simulink model "fen_ut"  (Simulink 8.1)
settings: Solver=FixedStepDiscrete  StartTime=0.0  StopTime=Inf  FixedStep=0.005  RelTol=1e-3
libraries: fen x1
settings Model: Creator=xsellart  LastModifiedBy=AT015555
settings DataIOCC: SignalLoggingSaveFormat=Dataset
settings OptimizationCC: ExpressionDepthLimit=128
settings DebuggingCC: FcnCallInpInsideContextMsg=EnableAllAsError
settings GRTTargetCC: CombineOutputUpdateFcns=on  GRTInterface=off

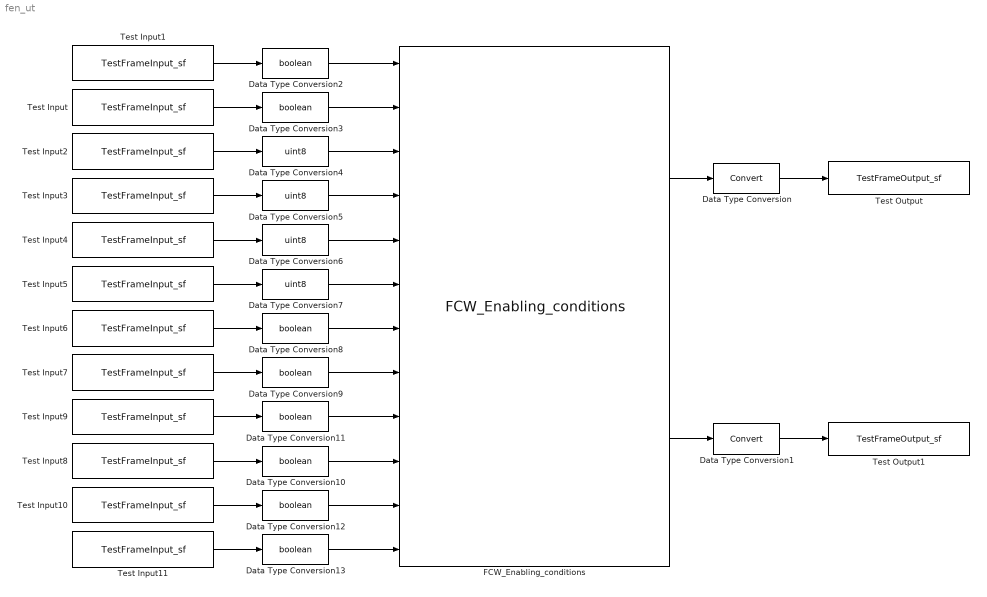
== system fen_ut ==
  Data Type Conversion : DataTypeConversion
  Data Type Conversion1 : DataTypeConversion
  Data Type Conversion{2..3,8..13} (8 alike) : DataTypeConversion  OutDataTypeStr=boolean
  Data Type Conversion{4..7} (4 alike) : DataTypeConversion  OutDataTypeStr=uint8
  FCW_Enabling_conditions : fen/FCW_Enabling_conditions
  Test Input : S-Function  FunctionName=TestFrameInput_sf  Parameters=varname,sampletime  EnableBusSupport=off  mask(Test Input){varname=VDINR_FCWEnableO_flg, sampletime=0.005}
      mask prompts: varname "Name:"; sampletime "Sample Time:"
      mask help: Outputs the value of a Test Input variable from an Excel spreadsheet when used with the runsiltest script. Otherwise outputs 0.
      mask Display: fprintf('Test Input:\n%s',varname);
  Test Input1 : S-Function  FunctionName=TestFrameInput_sf  Parameters=varname,sampletime  EnableBusSupport=off  mask(Test Input){varname=VDINR_FCWEnableH_flg, sampletime=0.005}
      mask prompts: varname "Name:"; sampletime "Sample Time:"
      mask help: Outputs the value of a Test Input variable from an Excel spreadsheet when used with the runsiltest script. Otherwise outputs 0.
      mask Display: fprintf('Test Input:\n%s',varname);
  Test Input10 : S-Function  FunctionName=TestFrameInput_sf  Parameters=varname,sampletime  EnableBusSupport=off  mask(Test Input){varname=VDHP_DisableADASFun_flg, sampletime=0.005}
      mask prompts: varname "Name:"; sampletime "Sample Time:"
      mask help: Outputs the value of a Test Input variable from an Excel spreadsheet when used with the runsiltest script. Otherwise outputs 0.
      mask Display: fprintf('Test Input:\n%s',varname);
  Test Input11 : S-Function  FunctionName=TestFrameInput_sf  Parameters=varname,sampletime  EnableBusSupport=off  mask(Test Input){varname=VDHP_DisableFCW_flg, sampletime=0.005}
      mask prompts: varname "Name:"; sampletime "Sample Time:"
      mask help: Outputs the value of a Test Input variable from an Excel spreadsheet when used with the runsiltest script. Otherwise outputs 0.
      mask Display: fprintf('Test Input:\n%s',varname);
  Test Input2 : S-Function  FunctionName=TestFrameInput_sf  Parameters=varname,sampletime  EnableBusSupport=off  mask(Test Input){varname=VDINR_KeySwitchStatus_enum, sampletime=0.005}
      mask prompts: varname "Name:"; sampletime "Sample Time:"
      mask help: Outputs the value of a Test Input variable from an Excel spreadsheet when used with the runsiltest script. Otherwise outputs 0.
      mask Display: fprintf('Test Input:\n%s',varname);
  Test Input3 : S-Function  FunctionName=TestFrameInput_sf  Parameters=varname,sampletime  EnableBusSupport=off  mask(Test Input){varname=VPER_CameraStatus_enum, sampletime=0.005}
      mask prompts: varname "Name:"; sampletime "Sample Time:"
      mask help: Outputs the value of a Test Input variable from an Excel spreadsheet when used with the runsiltest script. Otherwise outputs 0.
      mask Display: fprintf('Test Input:\n%s',varname);
  Test Input4 : S-Function  FunctionName=TestFrameInput_sf  Parameters=varname,sampletime  EnableBusSupport=off  mask(Test Input){varname=VPER_RadarStatus_enum, sampletime=0.005}
      mask prompts: varname "Name:"; sampletime "Sample Time:"
      mask help: Outputs the value of a Test Input variable from an Excel spreadsheet when used with the runsiltest script. Otherwise outputs 0.
      mask Display: fprintf('Test Input:\n%s',varname);
  Test Input5 : S-Function  FunctionName=TestFrameInput_sf  Parameters=varname,sampletime  EnableBusSupport=off  mask(Test Input){varname=VPER_FusionStatus_enum, sampletime=0.005}
      mask prompts: varname "Name:"; sampletime "Sample Time:"
      mask help: Outputs the value of a Test Input variable from an Excel spreadsheet when used with the runsiltest script. Otherwise outputs 0.
      mask Display: fprintf('Test Input:\n%s',varname);
  Test Input6 : S-Function  FunctionName=TestFrameInput_sf  Parameters=varname,sampletime  EnableBusSupport=off  mask(Test Input){varname=VIFO_VehicleStatusOk_flg, sampletime=0.005}
      mask prompts: varname "Name:"; sampletime "Sample Time:"
      mask help: Outputs the value of a Test Input variable from an Excel spreadsheet when used with the runsiltest script. Otherwise outputs 0.
      mask Display: fprintf('Test Input:\n%s',varname);
  Test Input7 : S-Function  FunctionName=TestFrameInput_sf  Parameters=varname,sampletime  EnableBusSupport=off  mask(Test Input){varname=VDINR_HMICANValid_flg, sampletime=0.005}
      mask prompts: varname "Name:"; sampletime "Sample Time:"
      mask help: Outputs the value of a Test Input variable from an Excel spreadsheet when used with the runsiltest script. Otherwise outputs 0.
      mask Display: fprintf('Test Input:\n%s',varname);
  Test Input8 : S-Function  FunctionName=TestFrameInput_sf  Parameters=varname,sampletime  EnableBusSupport=off  mask(Test Input){varname=VIFO_DriverSafetyStatusOk_flg, sampletime=0.005}
      mask prompts: varname "Name:"; sampletime "Sample Time:"
      mask help: Outputs the value of a Test Input variable from an Excel spreadsheet when used with the runsiltest script. Otherwise outputs 0.
      mask Display: fprintf('Test Input:\n%s',varname);
  Test Input9 : S-Function  FunctionName=TestFrameInput_sf  Parameters=varname,sampletime  EnableBusSupport=off  mask(Test Input){varname=VDHP_DisableDBS_flg, sampletime=0.005}
      mask prompts: varname "Name:"; sampletime "Sample Time:"
      mask help: Outputs the value of a Test Input variable from an Excel spreadsheet when used with the runsiltest script. Otherwise outputs 0.
      mask Display: fprintf('Test Input:\n%s',varname);
  Test Output : S-Function  FunctionName=TestFrameOutput_sf  Parameters=varname,sampletime  EnableBusSupport=off  mask(Test Output){varname=VJUD_FCWEnableReq_flg, sampletime=-1}
      mask prompts: varname "Name:"; sampletime "Sample Time:"
      mask help: Samples the value of a Test Output variable from an Excel spreadsheet when used with the runsiltest script. Otherwise does nothing.
      mask Display: fprintf('Test Output:\n%s',varname);
  Test Output1 : S-Function  FunctionName=TestFrameOutput_sf  Parameters=varname,sampletime  EnableBusSupport=off  mask(Test Output){varname=VJUD_FCWDBSAllowed_flg, sampletime=-1}
      mask prompts: varname "Name:"; sampletime "Sample Time:"
      mask help: Samples the value of a Test Output variable from an Excel spreadsheet when used with the runsiltest script. Otherwise does nothing.
      mask Display: fprintf('Test Output:\n%s',varname);
  wires:
  FCW_Enabling_conditions/1 -> Data Type Conversion/1
  Data Type Conversion/1 -> Test Output/1
  FCW_Enabling_conditions/2 -> Data Type Conversion1/1
  Data Type Conversion1/1 -> Test Output1/1
  Test Input1/1 -> Data Type Conversion2/1
  Data Type Conversion2/1 -> FCW_Enabling_conditions/1
  Test Input/1 -> Data Type Conversion3/1
  Data Type Conversion3/1 -> FCW_Enabling_conditions/2
  Test Input2/1 -> Data Type Conversion4/1
  Data Type Conversion4/1 -> FCW_Enabling_conditions/3
  Test Input3/1 -> Data Type Conversion5/1
  Data Type Conversion5/1 -> FCW_Enabling_conditions/4
  Test Input4/1 -> Data Type Conversion6/1
  Data Type Conversion6/1 -> FCW_Enabling_conditions/5
  Test Input5/1 -> Data Type Conversion7/1
  Test Input6/1 -> Data Type Conversion8/1
  Data Type Conversion8/1 -> FCW_Enabling_conditions/7
  Test Input7/1 -> Data Type Conversion9/1
  Data Type Conversion9/1 -> FCW_Enabling_conditions/8
  Test Input9/1 -> Data Type Conversion11/1
  Data Type Conversion11/1 -> FCW_Enabling_conditions/9
  Data Type Conversion7/1 -> FCW_Enabling_conditions/6
  Test Input8/1 -> Data Type Conversion10/1
  Data Type Conversion10/1 -> FCW_Enabling_conditions/10
  Test Input10/1 -> Data Type Conversion12/1
  Data Type Conversion12/1 -> FCW_Enabling_conditions/11
  Test Input11/1 -> Data Type Conversion13/1
  Data Type Conversion13/1 -> FCW_Enabling_conditions/12
